simulink model "Book6332"  (R2019b)
settings: Solver=ode4  StartTime=0.0  StopTime=20  FixedStep=0.001  RelTol=1e-3
settings Model: Creator=user  LastModifiedBy=user

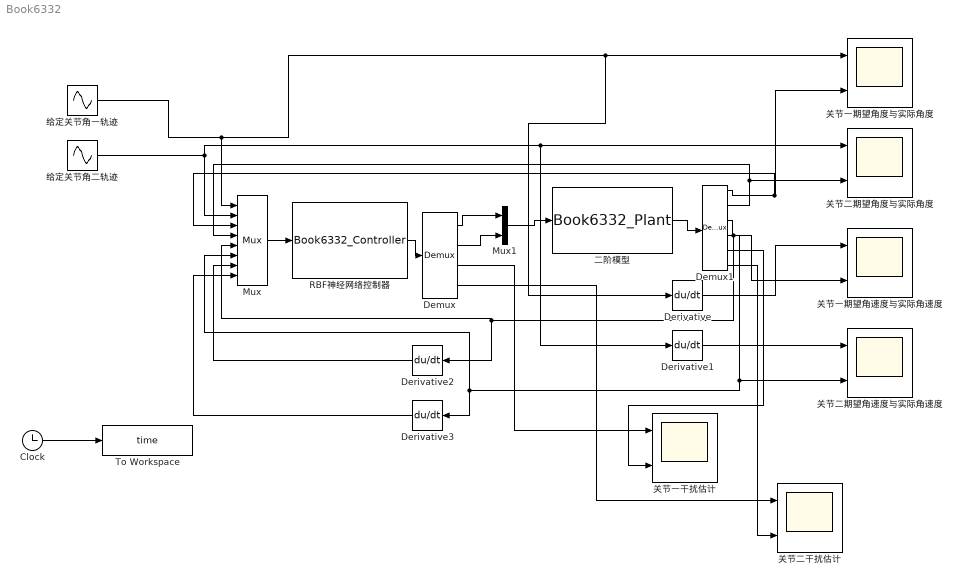
== system Book6332 ==
  Clock : Clock
  Demux : Demux
  Demux1 : Demux  Outputs=6
  Derivative{,1..3} (4 alike) : Derivative
  Mux : Mux  Inputs=8
  Mux1 : Mux  Inputs=2
  RBF神经网络控制器 : S-Function  FunctionName=Book6332_Controller  SFunctionDeploymentMode=off  EnableBusSupport=off
  To Workspace : ToWorkspace  VariableName=time  SaveFormat=Timeseries  SampleTime=-1
  二阶模型 : S-Function  FunctionName=Book6332_Plant  SFunctionDeploymentMode=off  EnableBusSupport=off
  关节一干扰估计 : Scope  NumInputPorts=2
  关节一期望角度与实际角度 : Scope  NumInputPorts=2
  关节一期望角速度与实际角速度 : Scope  NumInputPorts=2
  关节二干扰估计 : Scope  NumInputPorts=2
  关节二期望角度与实际角度 : Scope  NumInputPorts=2
  关节二期望角速度与实际角速度 : Scope  NumInputPorts=2
  给定关节角一轨迹 : Sin  SampleTime=0
  给定关节角二轨迹 : Sin  SampleTime=0
  wires:
  Demux1/3 -> Derivative2/1, Mux/5, 关节一期望角速度与实际角速度/2
  Demux/3 -> 关节一干扰估计/1
  给定关节角二轨迹/1 -> Mux/2, 关节二期望角度与实际角度/1, Derivative1/1
  给定关节角一轨迹/1 -> Derivative/1, 关节一期望角度与实际角度/1, Mux/1
  Derivative1/1 -> 关节二期望角速度与实际角速度/1
  Demux/1 -> Mux1/1
  Derivative/1 -> 关节一期望角速度与实际角速度/1
  Mux1/1 -> 二阶模型/1
  Demux/2 -> Mux1/2
  Clock/1 -> To Workspace/1
  Demux1/1 -> Mux/3, 关节一期望角度与实际角度/2
  二阶模型/1 -> Demux1/1
  RBF神经网络控制器/1 -> Demux/1
  Demux1/2 -> Mux/4, 关节二期望角度与实际角度/2
  Mux/1 -> RBF神经网络控制器/1
  Demux1/4 -> 关节二期望角速度与实际角速度/2, Derivative3/1, Mux/6
  Demux/4 -> 关节二干扰估计/1
  Derivative2/1 -> Mux/7
  Derivative3/1 -> Mux/8
  Demux1/5 -> 关节一干扰估计/2
  Demux1/6 -> 关节二干扰估计/2
